simulink model "Assignment2"  (R2020b)
settings: Solver=VariableStepAuto  StartTime=0.0  StopTime=10  RelTol=1e-3
values from neighbouring files (symbols this model uses):
  J = 1.2e-2    (= 0.012)    [Assignment1.m]    (also in Assignment2.m = 2; dSpaceLab.m = 4.69391617652e-05)
  Kf = 0.25    [Assignment2.m]
  L_M = 0.1    [Assignment2.m]
  Ld = 1*10^-3    (= 0.001)    [Assignment2.m]
  Lq = 1*10^-3    (= 0.001)    [Assignment2.m]
  R = 1.9    [Assignment1.m]    (also in Assignment2.m = 1.5)
settings Model: Creator=sebastian  LastModifiedBy=sebastian

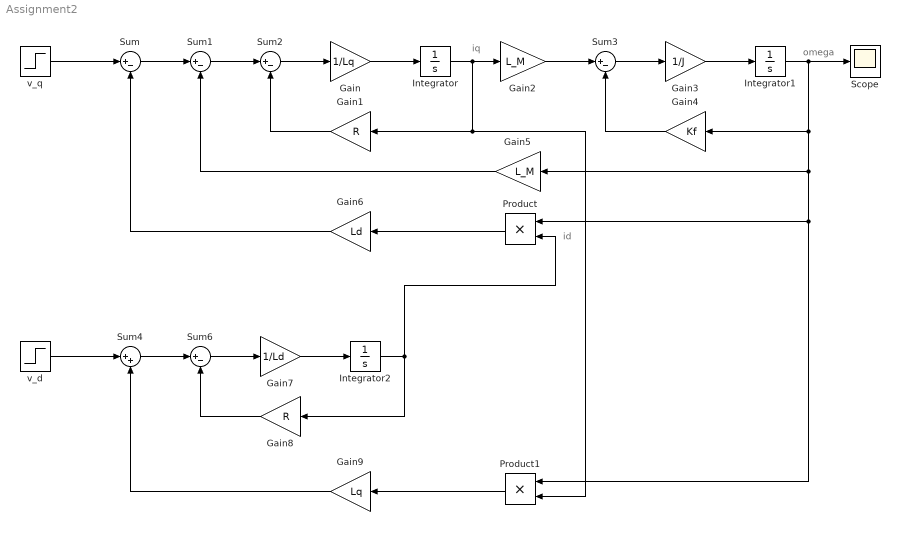
== system Assignment2 ==
  note: iq
  note: id
  note: omega
  Gain : Gain  Gain=1/Lq
  Gain1 : Gain  Gain=R
  Gain2 : Gain  Gain=L_M
  Gain3 : Gain  Gain=1/J
  Gain4 : Gain  Gain=Kf
  Gain5 : Gain  Gain=L_M
  Gain6 : Gain  Gain=Ld
  Gain7 : Gain  Gain=1/Ld
  Gain8 : Gain  Gain=R
  Gain9 : Gain  Gain=Lq
  Integrator : Integrator
  Integrator1 : Integrator
  Integrator2 : Integrator
  Product : Product
  Product1 : Product
  Scope : Scope
  Sum{,1..3,6} (5 alike) : Sum  Inputs=|+-
  Sum4 : Sum  Inputs=|++
  v_d : Step  After=10  SampleTime=0
  v_q : Step  After=10  SampleTime=0
  wires:
  v_q/1 -> Sum/1
  Sum/1 -> Sum1/1
  Sum1/1 -> Sum2/1
  Sum2/1 -> Gain/1
  Gain/1 -> Integrator/1
  Integrator/1 -> Gain2/1, Product1/2, Gain1/1
  Gain1/1 -> Sum2/2
  Gain2/1 -> Sum3/1
  Sum3/1 -> Gain3/1
  Gain3/1 -> Integrator1/1
  Integrator1/1 -> Scope/1, Product1/1, Product/1, Gain5/1, Gain4/1
  Gain4/1 -> Sum3/2
  Gain5/1 -> Sum1/2
  Gain6/1 -> Sum/2
  Product/1 -> Gain6/1
  v_d/1 -> Sum4/1
  Sum6/1 -> Gain7/1
  Gain7/1 -> Integrator2/1
  Integrator2/1 -> Gain8/1, Product/2
  Gain8/1 -> Sum6/2
  Sum4/1 -> Sum6/1
  Product1/1 -> Gain9/1
  Gain9/1 -> Sum4/2
